simulink model "PID_model"  (R2015a)
settings: Solver=ode45  StartTime=0.0  StopTime=3000
values from neighbouring files (symbols this model uses):
  A = [0 1; -K/M -rho/M]    [noSaturation.m]    (also in saturation.m)
  B = [0; 1]    [noSaturation.m]    (also in saturation.m)
  C = [1 0]    [noSaturation.m]    (also in saturation.m)
  D = 0    [noSaturation.m]    (also in saturation.m)
  k_d = 1.6    [noSaturation.m]    (also in saturation.m)
  k_i = 2    [noSaturation.m]    (also in saturation.m = 0.6)
  k_p = 1.5    [noSaturation.m]    (also in saturation.m = 0.5)
  xr = 4    [noSaturation.m]    (also in saturation.m)
settings Model: Creator=nightstalker  LastModifiedBy=nightstalker
settings SolverCC: MaxConsecutiveMinStep=10

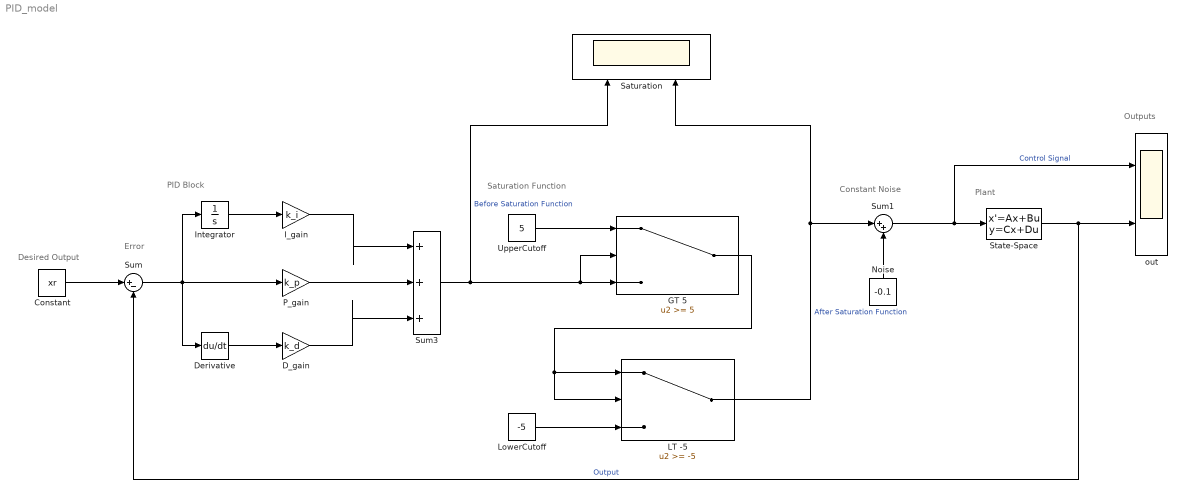
== system PID_model ==
  note: Error
  note: Outputs
  note: Plant
  note: Desired Output
  note: PID Block
  note: Constant Noise
  note: Saturation Function
  Constant : Constant  Value=xr
  D_gain : Gain  Gain=k_d
  Derivative : Derivative  CoefficientInTFapproximation=1
  GT 5 : Switch  Threshold=5  ZeroCross=off
  I_gain : Gain  Gain=k_i
  Integrator : Integrator
  LT -5 : Switch  Threshold=-5  ZeroCross=off
  LowerCutoff : Constant  Value=-5
  Noise : Constant  Value=-0.1
  P_gain : Gain  Gain=k_p
  Saturation : Scope  NumInputPorts=2
      settings: YMin=-5~-5  YMax=5~5
  State-Space : StateSpace  A=A  B=B  C=C  D=D  X0=0
  Sum : Sum  Inputs=|+-
  Sum1 : Sum  Inputs=|++
  Sum3 : Sum  Inputs=|+++|
  UpperCutoff : Constant  Value=5
  out : Scope  NumInputPorts=2
      settings: YMin=-5~-5  YMax=5~5
  wires:
  Integrator/1 -> I_gain/1
  Sum/1 -> P_gain/1, Derivative/1, Integrator/1
  Derivative/1 -> D_gain/1
  Constant/1 -> Sum/1
  D_gain/1 -> Sum3/3
  P_gain/1 -> Sum3/2
  I_gain/1 -> Sum3/1
  State-Space/1 -> Sum/2, out/2  "Output"
  Noise/1 -> Sum1/2
  Sum1/1 -> State-Space/1, out/1  "Control Signal"
  GT 5/1 -> LT -5/2, LT -5/1
  UpperCutoff/1 -> GT 5/1
  LowerCutoff/1 -> LT -5/3
  Sum3/1 -> GT 5/3, GT 5/2, Saturation/1  "Before Saturation Function"
  LT -5/1 -> Sum1/1, Saturation/2  "After Saturation Function"
